simulink library "GRC_Lib"  (R2017b)
settings: Solver=VariableStepAuto  StartTime=0.0  StopTime=10.0  RelTol=1e-3  EnableMultiTasking=on
StartFcn:
  | set_param('AdvancedOperations','ZoomFactor','100');
undefined symbols (not defined in the file): Test
libraries: GRC_Lib x203, simulink x1
(part 1 of 4)
settings Model: Creator=Administrator  LastModifiedBy=WangYunHao
settings DataIOCC: LimitDataPoints=on
settings OptimizationCC: LifeSpan=inf
settings DebuggingCC: AllowSymbolicDim=off  SFUnexpectedBacktrackingDiag=warning  SFNoUnconditionalDefaultTransitionDiag=warning  SFExecutionAtInitializationDiag=none
settings ModelReferenceCC: PropagateSignalLabelsOutOfModel=off
settings CodeAppCC: StateflowObjectComments=on
settings GRTTargetCC: TargetLangStandard=C89/C90 (ANSI)
settings ConfigComp: CovMetricSettings=dw  CovHtmlReporting=on  CovSaveCumulativeToWorkspaceVar=on  CovSaveSingleToWorkspaceVar=on  CovExternalEMLEnable=off

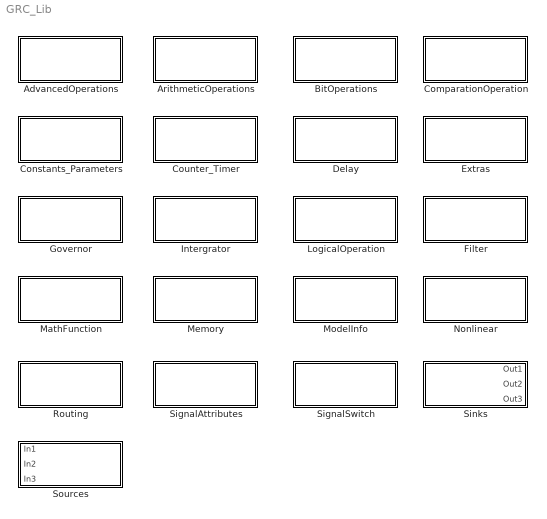
== system GRC_Lib ==
  AdvancedOperations : Subsystem
  ArithmeticOperations : Subsystem
  BitOperations : Subsystem
  ComparationOperation : Subsystem
  Constants_Parameters : Subsystem
  Counter_Timer : Subsystem
  Delay : Subsystem
  Extras : Subsystem
  Filter : Subsystem
  Governor : Subsystem
  Intergrator : Subsystem
  LogicalOperation : Subsystem
  MathFunction : Subsystem
  Memory : Subsystem
  ModelInfo : Subsystem
  Nonlinear : Subsystem
  Routing : Subsystem
  SignalAttributes : Subsystem
  SignalSwitch : Subsystem
  Sinks : Subsystem
  Sources : Subsystem

== system GRC_Lib/AdvancedOperations ==
  note: // What's the 2D length function
      | and lookup methods???
  note: // What's the 1D Length function?
  1D_DynamicLookupTable : Subsystem  TreatAsAtomicUnit=on  mask{method=Use Input Nearest, IpDTx=int8, IpDTy=single, OpDT=single, Length1D=50}
      mask prompts: method "Lookup Method"; IpDTx "xData Datatype"; IpDTy "yData Datatype"; OpDT "Output Data Type"; Length1D "1D Table Length (Min. 2 Max. 200)"
      mask init:
      | %%% Input port number detection 
      | if isequal(str2num(get_param(gcb,'Length1D')),[])
      |     if Length1D<2
      |         error('*** ERROR_11 ***    1D Table Length must belong to [2,200].');
      |     elseif Length1D>200
      |         error('*** ERROR_12 ***    1D Table Length must belong to [2,200].');
      |     else
      |     end
      | else
      |     Lgth = str2num(get_param(gcb,'Length1D'));
      |     if Lgth<2
      |         error('*** ERROR_21 ***    1D Table Length must belong to [2,200].');
      |     elseif Lgth>200
      |         error('*** ERROR_22 ***    1D Table Length must belong to [2,200].');
      |     else
      |     end
      | end
      | 
      | set_param([gcb '/Dynamic1D'],'OutDataTypeStr',OpDT);
      | MethDtr = get_param(gcb,'method');
      | set_param([gcb '/Dynamic1D'], 'LookUpMeth',MethDtr);
      | 
      | DTStry = get_param(gcb,'OpDT');
      | try
      |     if isequal(DTStry,'boolean')
      |         FColor = '[0.901961, 0.313725, 0.078431]'; 
      |     elseif isequal(DTStry,'double')||isequal(DTStry,'single')
      |         FColor = '[0.313725, 0.117647, 0.352941]';  
      |     else
      |         FColor = '[0.196078, 0.549020, 0.549020]';
      |     end        
      | catch
      | end
      | set_param([gcb '/y'],'ForegroundColor',FColor);
      | set_param(gcb,'ForegroundColor',FColor);
      settings: AttributesFormatString=Length = %<Length1D>
      mask TypeOptions method: Interpolation-Use End Values | Use Input Nearest | Use Input Below | Use Input Above
      mask Callback Length1D:
      | % %%% Input port number detection
      | % if isequal(str2num(get_param(gcb,'Length1D')),[])
      | %    error('*** ERROR_1 ***    1D Table Length can not be a %s.',class(get_param(gcb,'Length1D')));
      | % elseif str2num(get_param(gcb,'Length1D'))<2
      | %    error('*** ERROR_2 ***    1D Table Length must belong to [2,200].');
      | % elseif str2num(get_param(gcb,'Length1D'))>200
      | %    error('*** ERROR_2 ***    1D Table Length must belong to [2,200].');
      | % else
      | % end
      mask Display:
      | color('green');
      | disp ('Dynamic\nLookup Table\n(1D)');
  1D_LookupTableContrafunctional : Subsystem
      mask Display:
      | color('green');
      | disp (sprintf('LookupTable\nContrafunctional\n(1D)'));
  2D_DynamicLookupTable : Subsystem  TreatAsAtomicUnit=on  mask{method=Interpolation-Use End Values, Lengthx=10, Lengthy=10, IpDTx=int8, IpDTy=single, IpDTm=int16, MrDT=double, OpDT=double}
      mask prompts: method "Lookup Method"; Lengthx "x Axis Length (Min. 2 Max. 50)"; Lengthy "y Axis Length (Min. 2 Max. 50)"; IpDTx "xData Datatype"; IpDTy "yData Datatype"; IpDTm "mData Datatype"; MrDT "Intermediate Results Data Type"; OpDT "Output Data Type"
      mask init:
      | %%% Input Lentghx number detection
      | if isequal(str2num(get_param(gcb,'Lengthx')),[])
      |     if Lengthx<2
      |         error('*** ERROR_x11 ***    x Axis Length must belong to [2,50].');
      |     elseif Lengthx>50
      |         error('*** ERROR_x12 ***    x Axis Length must belong to [2,50].');
      |     else
      |     end
      | else 
      |     Lgthx = str2num(get_param(gcb,'Lengthx'));
      |     if Lgthx<2
      |         error('*** ERROR_x21 ***    x Axis Length must belong to [2,50].');
      |     elseif Lgthx>50
      |         error('*** ERROR_x22 ***    x Axis Length must belong to [2,50].');
      |     else
      |     end
      | end
      | %%% Input Lentghy number detection
      | if isequal(str2num(get_param(gcb,'Lengthy')),[])
      |     if Lengthy<2
      |         error('*** ERROR_y11 ***    y Axis Length must belong to [2,50].');
      |     elseif Lengthy>50
      |         error('*** ERROR_y12 ***    y Axis Length must belong to [2,50].');
      |     else
      |     end
      | else 
      |     Lgthy = str2num(get_param(gcb,'Lengthy'));
      |     if Lgthy<2
      |         error('*** ERROR_y21 ***    y Axis Length must belong to [2,50].');
      |     elseif Lgthy>50
      |         error('*** ERROR_y22 ***    y Axis Length must belong to [2,50].');
      |     else
      |     end
      | end
      | %%%%%%%%%%%%%%%%%%%%%%%%%%%%%%%%%%%%%%%%%%%%%%%%%%%%%%%%%%%%%%%%%%%%%%%%%%%
      | DTStrM = get_param(gcb,'MrDT');
      | DTStrO = get_param(gcb,'OpDT');
      | set_param([gcb '/Dynamic2D'],'IntermediateResultsDataTypeStr',DTStrM);
      | set_param([gcb '/Dynamic2D'],'OutDataTypeStr',DTStrO);
      | 
      | try
      |     if isequal(DTStrO,'boolean')
      |         FColor = '[0.901961, 0.313725, 0.078431]'; 
      |     elseif isequal(DTStrO,'double')||isequal(DTStrO,'single')
      |         FColor = '[0.313725, 0.117647, 0.352941]';  
      |     else
      |         FColor = '[0.196078, 0.549020, 0.549020]';
      |     end        
      | catch
      | end
      | set_param([gcb '/out'],'ForegroundColor',FColor);
      | set_param(gcb,'ForegroundColor',FColor);
      settings: AttributesFormatString=|
      | xData Length = %<Lengthx>
      | yData Length = %<Lengthy>
      mask TypeOptions method: Interpolation-Use End Values | Use Input Below
      mask Callback Lengthx:
      | % %%% Input port number detection
      | % if isequal(str2num(get_param(gcb,'Lengthx')),[])
      | %    error('*** ERROR_1 ***    x Axis Length can not be a %s.',class(get_param(gcb,'Lengthx')));
      | % elseif str2num(get_param(gcb,'Lengthx'))<2
      | %    error('*** ERROR_2 ***    x Axis Length must belong to [2,50].');
      | % elseif str2num(get_param(gcb,'Lengthx'))>50
      | %    error('*** ERROR_2 ***    x Axis Length must belong to [2,50].');
      | % else
      | % end
      mask Callback Lengthy:
      | % %%% Input port number detection
      | % if isequal(str2num(get_param(gcb,'Lengthy')),[])
      | %    error('*** ERROR_1 ***    y Axis Length can not be a %s.',class(get_param(gcb,'Lengthy')));
      | % elseif str2num(get_param(gcb,'Lengthy'))<2
      | %    error('*** ERROR_2 ***    y Axis Length must belong to [2,50].');
      | % elseif str2num(get_param(gcb,'Lengthy'))>50
      | %    error('*** ERROR_2 ***    y Axis Length must belong to [2,50].');
      | % else
      | % end
      mask Display:
      | color('green');
      | disp (sprintf('Dynamic\nLookup Table\n(2D)'));
  DynAvrgFltr : Subsystem  TreatAsAtomicUnit=on  mask{IpDT=single, RngSizeMsk=5}
      mask prompts: IpDT "Input Data Type"; RngSizeMsk "Dynamic Average Filter Step (Min 1, Max 200)"
      mask init:
      | %%% Input port number detection 
      | if isequal(str2num(get_param(gcb,'RngSizeMsk')),[])
      |     if RngSizeMsk<1
      |         error('*** ERROR_11 ***    Dynamic Average Filter Step must belong to [1,200].');
      |     elseif RngSizeMsk>200
      |         error('*** ERROR_12 ***    Dynamic Average Filter Step must belong to [1,200].');
      |     else
      |     end
      | else
      |     RgSiz = str2num(get_param(gcb,'RngSizeMsk'));
      |     if RgSiz<1
      |         error('*** ERROR_21 ***    Dynamic Average Filter Step must belong to [1,200].');
      |     elseif RgSiz>200
      |         error('*** ERROR_22 ***    Dynamic Average Filter Step must belong to [1,200].');
      |     else
      |     end
      | end
      | 
      | RngSize = RngSizeMsk;
      | DTStr = get_param(gcb,'IpDT');
      | set_param([gcb '/Constant6'],'OutDataTypeStr',DTStr);
      | set_param([gcb '/SUB'],'IpDT',DTStr);
      | set_param([gcb '/DIV'],'IpDT',DTStr);
      | set_param([gcb '/SUM1'],'IpDT',DTStr);
      | 
      | DTStry = get_param([gcb '/SUM1/Sum1'],'OutDataTypeStr');
      | try
      |     if isequal(DTStry,'boolean')
      |         FColor = '[0.901961, 0.313725, 0.078431]'; 
      |     elseif isequal(DTStry,'double')||isequal(DTStry,'single')
      |         FColor = '[0.313725, 0.117647, 0.352941]';  
      |     else
      |         FColor = '[0.196078, 0.549020, 0.549020]';
      |     end        
      | catch
      | end
      | set_param([gcb '/out'],'ForegroundColor',FColor);
      | set_param(gcb,'ForegroundColor',FColor);
      settings: AttributesFormatString=%<RngSizeMsk>
      mask Callback RngSizeMsk:
      | % %%% Input port number detection
      | % if str2num(get_param(gcb,'RngSizeMsk'))<1
      | %    error('*** ERROR ***    Dynamic Average Filter Step must belong to [1,200].');
      | % elseif str2num(get_param(gcb,'RngSizeMsk'))>200
      | %    error('*** ERROR ***    Dynamic Average Filter Step must belong to [1,200].');
      | % else
      | % end
      mask Display:
      | % color('green');
      | % disp ('DynAvrgFltr');
      | image('DynAvrgFltr.jpg');
  VrblTmDelay : Subsystem  TreatAsAtomicUnit=on  mask{IpDTT=double, IpDTu=boolean, MaxBufferMsk=2000, IniVal=0}
      mask prompts: IpDTT "Input T Data Type"; IpDTu "Input u Data Type"; MaxBufferMsk "Maximum Buffer Size (Max 2000)"; IniVal "Initial Value"
      mask init:
      | %%% Input port number detection 
      | if isequal(str2num(get_param(gcb,'MaxBufferMsk')),[])
      |     if MaxBufferMsk<2
      |         error('*** ERROR_11 ***    Maximum Buffer Size must belong to [2,2000].');
      |     elseif MaxBufferMsk>2000
      |         error('*** ERROR_12 ***    Maximum Buffer Size must belong to [2,2000].');
      |     else
      |     end
      | else
      |     MxBf = str2num(get_param(gcb,'MaxBufferMsk'));
      |     if MxBf<2
      |         error('*** ERROR_21 ***    Maximum Buffer Size must belong to [2,2000].');
      |     elseif MxBf>2000
      |         error('*** ERROR_22 ***    Maximum Buffer Size must belong to [2,2000].');
      |     else
      |     end
      | end
      | 
      | MaxBuffer = MaxBufferMsk;
      | initValue = IniVal;
      | DTStrT = get_param(gcb,'IpDTT');
      | set_param([gcb '/Constant'],'OutDataTypeStr',DTStrT);
      | set_param([gcb '/DIV'],'IpDT',DTStrT);
      | 
      | DTStryu = get_param(gcb,'IpDTu');
      | try
      |     if isequal(DTStryu,'boolean')
      |         FColor = '[0.901961, 0.313725, 0.078431]'; 
      |     elseif isequal(DTStryu,'double')||isequal(DTStryu,'single')
      |         FColor = '[0.313725, 0.117647, 0.352941]';  
      |     else
      |         FColor = '[0.196078, 0.549020, 0.549020]';
      |     end        
      | catch
      | end
      | set_param([gcb '/y'],'ForegroundColor',FColor);
      | set_param(gcb,'ForegroundColor',FColor);
      settings: AttributesFormatString=MaxBufferSize = %<MaxBufferMsk>
      mask Callback MaxBufferMsk:
      | % %%% Input port number detection
      | % if str2num(get_param(gcb,'MaxBufferMsk'))<2
      | %    error('*** ERROR ***    Maximum Buffer Size must belong to [2,2000].');
      | % elseif str2num(get_param(gcb,'MaxBufferMsk'))>2000
      | %    error('*** ERROR ***    Maximum Buffer Size must belong to [2,2000].');
      | % else
      | % end
      mask Display:
      | % color('green');
      | % disp ('VrblTmDelay');
      | % image('VrblTmDelay.jpg');
      | image(imread('VrblTmDelay.jpg'),[0.2,0.1,0.7,0.8]);

== system GRC_Lib/ArithmeticOperations ==
  DIV : Subsystem  TreatAsAtomicUnit=on  mask{MinDivVal=1e-15, IpDT=int8}
      mask prompts: MinDivVal "Minimum Allowed Divided Value"; IpDT "Input Data Type"
      mask init:
      | MinVal = MinDivVal;
      | set_param([gcb '/Constant1'],'OutDataTypeStr',IpDT);
      | set_param([gcb '/Divide'],'OutDataTypeStr',IpDT);
      | 
      | DTStry = get_param([gcb '/Divide'],'OutDataTypeStr');
      | try
      |     if isequal(DTStry,'boolean')
      |         FColor = '[0.901961, 0.313725, 0.078431]'; 
      |     elseif isequal(DTStry,'double')||isequal(DTStry,'single')
      |         FColor = '[0.313725, 0.117647, 0.352941]';  
      |     else
      |         FColor = '[0.196078, 0.549020, 0.549020]';
      |     end        
      | catch
      | end
      | set_param([gcb '/Out'],'ForegroundColor',FColor);
      | set_param(gcb,'ForegroundColor',FColor);
      mask Display:
      | color('green');
      | port_label('input',1,'\fontname{Courier New}\fontsize{16}\bf×','texmode','on');
      | port_label('input',2,'\fontname{Courier New}\fontsize{16}\bf÷','texmode','on');
  GAIN : Subsystem  mask(GAIN){K=20, IpDT=double, OFChk=on}
      mask prompts: K "Gain"; IpDT "Input Data Type"; OFChk "Consider Overflow/Underflow (Integers Only)"
      mask help:
      | GRC Library for Function Development
      | (c) GRC, 2016
      |
      | Multiply the input by a gain factor.
      mask init:
      | GAIN=K;
      | 
      | DTStr = get_param(gcb,'IpDT');
      | OFChkStr = get_param(gcb,'OFChk');
      | try
      | if isequal(OFChkStr,'1')
      |     if isequal(DTStr,'int8')||isequal(DTStr,'uint8')
      |         set_param([gcb '/Gain1'],'OutDataTypeStr','uint16'); 
      |     elseif isequal(DTStr,'int16')||isequal(DTStr,'uint16')
      |         set_param([gcb '/Gain1'],'OutDataTypeStr','uint32'); 
      |     elseif isequal(DTStr,'int32')||isequal(DTStr,'uint32')
      |         set_param([gcb '/Gain1'],'OutDataTypeStr','uint32'); 
      |     elseif isequal(DTStr,'double')
      |         set_param([gcb '/Gain1'],'OutDataTypeStr','double'); 
      |     elseif isequal(DTStr,'single')
      |         set_param([gcb '/Gain1'],'OutDataTypeStr','single');
      |     end
      | else
      |     set_param([gcb '/Gain1'],'OutDataTypeStr',DTStr);
      | end
      | catch
      | end
      | 
      | DTStry = get_param([gcb '/Gain1'],'OutDataTypeStr');
      | try
      |     if isequal(DTStry,'boolean')
      |         FColor = '[0.901961, 0.313725, 0.078431]'; 
      |     elseif isequal(DTStry,'double')||isequal(DTStry,'single')
      |         FColor = '[0.313725, 0.117647, 0.352941]';  
      |     else
      |         FColor = '[0.196078, 0.549020, 0.549020]';
      |     end        
      | catch
      | end
      | set_param([gcb '/Out1'],'ForegroundColor',FColor);
      | set_param(gcb,'ForegroundColor',FColor);
      settings: AttributesFormatString=K=%<K>
      mask Display:
      | color('green');
      | disp('\fontsize{10}\bfK','texmode','on');
  MUL : Subsystem  mask(MUL){IpDT=double, OFChk=on}
      mask prompts: IpDT "Input Data Type"; OFChk "Consider Overflow/Underflow (Integers Only)"
      mask help:
      | GRC Library for Function Development
      | (c) GRC, 2016
      |
      | Multiplies two inputs.
      mask init:
      | DTStr = get_param(gcb,'IpDT');
      | OFChkStr = get_param(gcb,'OFChk');
      | try
      | if isequal(OFChkStr,'1')
      |     if isequal(DTStr,'int8')||isequal(DTStr,'uint8')
      |         set_param([gcb '/Mul1'],'OutDataTypeStr','uint16'); 
      |     elseif isequal(DTStr,'int16')||isequal(DTStr,'uint16')
      |         set_param([gcb '/Mul1'],'OutDataTypeStr','uint32'); 
      |     elseif isequal(DTStr,'int32')||isequal(DTStr,'uint32')
      |         set_param([gcb '/Mul1'],'OutDataTypeStr','uint32'); 
      |     elseif isequal(DTStr,'double')
      |         set_param([gcb '/Mul1'],'OutDataTypeStr','double'); 
      |     elseif isequal(DTStr,'single')
      |         set_param([gcb '/Mul1'],'OutDataTypeStr','single');
      |     end
      | else
      |     set_param([gcb '/Mul1'],'OutDataTypeStr',DTStr);
      | end
      | catch
      | end
      | 
      | DTStry = get_param([gcb '/Mul1'],'OutDataTypeStr');
      | try
      |     if isequal(DTStry,'boolean')
      |         FColor = '[0.901961, 0.313725, 0.078431]'; 
      |     elseif isequal(DTStry,'double')||isequal(DTStry,'single')
      |         FColor = '[0.313725, 0.117647, 0.352941]';  
      |     else
      |         FColor = '[0.196078, 0.549020, 0.549020]';
      |     end        
      | catch
      | end
      | set_param([gcb '/Out1'],'ForegroundColor',FColor);
      | set_param(gcb,'ForegroundColor',FColor);
      mask Display:
      | color('green');
      | disp('\fontsize{14}\bf×','texmode','on');
  NEG : Subsystem  mask(NEG){DTNEG=double}
      mask prompts: DTNEG "Output Data Type"
      mask help:
      | GRC Library for Function Development
      | (c) GRC, 2016
      |
      | Negates the input signal.
      mask init:
      | dtneg=get_param(gcb,'DTNEG');
      | set_param([gcb '/Neg1'],'OutDataTypeStr',dtneg);
      | 
      | DTStry = get_param([gcb '/Neg1'],'OutDataTypeStr');
      | try
      |     if isequal(DTStry,'boolean')
      |         FColor = '[0.901961, 0.313725, 0.078431]'; 
      |     elseif isequal(DTStry,'double')||isequal(DTStry,'single')
      |         FColor = '[0.313725, 0.117647, 0.352941]';  
      |     else
      |         FColor = '[0.196078, 0.549020, 0.549020]';
      |     end        
      | catch
      | end
      | set_param([gcb '/Out1'],'ForegroundColor',FColor);
      | set_param(gcb,'ForegroundColor',FColor);
      mask Display:
      | color('green')
      | disp('\fontsize{10}\bf-1','texmode','on')
  SUB : Subsystem  mask(SUB){IpDT=double, OFChk=on}
      mask prompts: IpDT "Input Data Type"; OFChk "Consider Overflow/Underflow (Integers Only)"
      mask help:
      | GRC Library for Function Development
      | (c) GRC, 2016
      |
      | Subtract input 2 from input 1.
      |
      | Input must have the same data type.
      mask init:
      | DTStr = get_param(gcb,'IpDT');
      | OFChkStr = get_param(gcb,'OFChk');
      | try
      | if isequal(OFChkStr,'1')
      |     if isequal(DTStr,'int8')||isequal(DTStr,'uint8')
      |         set_param([gcb '/Sub1'],'OutDataTypeStr','uint16'); 
      |     elseif isequal(DTStr,'int16')||isequal(DTStr,'uint16')
      |         set_param([gcb '/Sub1'],'OutDataTypeStr','uint32'); 
      |     elseif isequal(DTStr,'int32')||isequal(DTStr,'uint32')
      |         set_param([gcb '/Sub1'],'OutDataTypeStr','uint32'); 
      |     elseif isequal(DTStr,'double')
      |         set_param([gcb '/Sub1'],'OutDataTypeStr','double'); 
      |     elseif isequal(DTStr,'single')
      |         set_param([gcb '/Sub1'],'OutDataTypeStr','single');
      |     end
      | else
      |     set_param([gcb '/Sub1'],'OutDataTypeStr',DTStr);
      | end
      | catch
      | end
      | 
      | DTStry = get_param([gcb '/Sub1'],'OutDataTypeStr');
      | try
      |     if isequal(DTStry,'boolean')
      |         FColor = '[0.901961, 0.313725, 0.078431]'; 
      |     elseif isequal(DTStry,'double')||isequal(DTStry,'single')
      |         FColor = '[0.313725, 0.117647, 0.352941]';  
      |     else
      |         FColor = '[0.196078, 0.549020, 0.549020]';
      |     end        
      | catch
      | end
      | set_param([gcb '/Out1'],'ForegroundColor',FColor);
      | set_param(gcb,'ForegroundColor',FColor);
      mask Display:
      | color('green');
      | port_label('input',1,'\fontname{Courier New}\fontsize{16}\bf+','texmode','on');
      | port_label('input',2,'\fontname{Courier New}\fontsize{16}\bf-','texmode','on');
  SUB_Uint : Subsystem  TreatAsAtomicUnit=on  mask{IpDT=uint8}
      mask prompts: IpDT "Input Data Type"
      mask init:
      | DTStr = get_param(gcb,'IpDT');
      | set_param([gcb '/Constant'],'OutDataTypeStr',DTStr);
      | 
      | DTStry = get_param([gcb '/Constant'],'OutDataTypeStr');
      | try
      |     if isequal(DTStry,'boolean')
      |         FColor = '[0.901961, 0.313725, 0.078431]'; 
      |     elseif isequal(DTStry,'double')||isequal(DTStry,'single')
      |         FColor = '[0.313725, 0.117647, 0.352941]';  
      |     else
      |         FColor = '[0.196078, 0.549020, 0.549020]';
      |     end        
      | catch
      | end
      | set_param([gcb '/Out'],'ForegroundColor',FColor);
      | set_param(gcb,'ForegroundColor',FColor);
      settings: AttributesFormatString=SUB_Uint
      mask Display:
      | color('blue');
      | port_label('input',1,'\fontname{Courier New}\fontsize{16}\bf+','texmode','on');
      | port_label('input',2,'\fontname{Courier New}\fontsize{16}\bf-','texmode','on');
  SUM : Subsystem  mask(SUM){IpDT=single, OFChk=on}
      mask prompts: IpDT "Input Data Type"; OFChk "Consider Overflow/Underflow (Integers Only)"
      mask help:
      | GRC Library for Function Development
      | (c) GRC, 2016
      |
      | Caculates the sum of two input values.
      |
      | Input must have the same data type.
      mask init:
      | DTStr = get_param(gcb,'IpDT');
      | OFChkStr = get_param(gcb,'OFChk');
      | try
      | if isequal(OFChkStr,'1')
      |     if isequal(DTStr,'int8')||isequal(DTStr,'uint8')
      |         set_param([gcb '/Sum1'],'OutDataTypeStr','uint16');
      |     elseif isequal(DTStr,'int16')||isequal(DTStr,'uint16')
      |         set_param([gcb '/Sum1'],'OutDataTypeStr','uint32');
      |     elseif isequal(DTStr,'int32')||isequal(DTStr,'uint32')
      |         set_param([gcb '/Sum1'],'OutDataTypeStr','uint32'); 
      |     elseif isequal(DTStr,'double')
      |         set_param([gcb '/Sum1'],'OutDataTypeStr','double'); 
      |     elseif isequal(DTStr,'single')
      |         set_param([gcb '/Sum1'],'OutDataTypeStr','single');
      |     end
      | else
      |     set_param([gcb '/Sum1'],'OutDataTypeStr',DTStr);
      | end
      | catch
      | end
      | 
      | DTStry = get_param([gcb '/Sum1'],'OutDataTypeStr');
      | try
      |     if isequal(DTStry,'boolean')
      |         FColor = '[0.901961, 0.313725, 0.078431]'; 
      |     elseif isequal(DTStry,'double')||isequal(DTStry,'single')
      |         FColor = '[0.313725, 0.117647, 0.352941]';  
      |     else
      |         FColor = '[0.196078, 0.549020, 0.549020]';
      |     end        
      | catch
      | end
      | set_param([gcb '/Out1'],'ForegroundColor',FColor);
      | set_param(gcb,'ForegroundColor',FColor);
      mask Display:
      | color('green')
      | port_label('input',1,'\fontname{Courier New}\fontsize{16}\bf+','texmode','on')
      | port_label('input',2,'\fontname{Courier New}\fontsize{16}\bf+','texmode','on')

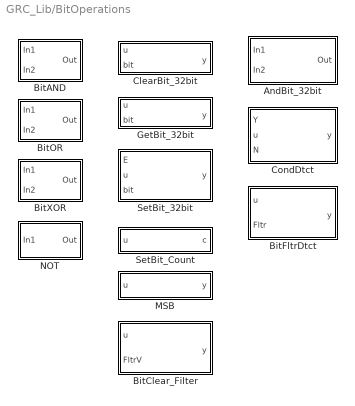
== system GRC_Lib/BitOperations ==
  AndBit_32bit : Subsystem  TreatAsAtomicUnit=on
      mask help:
      | This block judge whether at least one bit is set or not. If any bits are set, output is boolean 1, otherwise output is boolean 0.
      |
      | input 1 and input 2 should have same data type, and output is boolean.
      mask init:
      | FColor = '[0.901961, 0.313725, 0.078431]'; 
      | try
      |     set_param([gcb '/Out'],'ForegroundColor',FColor);
      |     set_param(gcb,'ForegroundColor',FColor);
      | catch
      | end
      mask Display:
      | % color('red');
      | % disp ('AndBit\n(8|16|32bit)');
      | image(imread('AndBit_32bit.jpg'),[0.03,0.1,0.95,0.8]);
  BitAND : Subsystem  TreatAsAtomicUnit=on  mask{IpDT=uint8}
      mask prompts: IpDT "Input Data Type"
      mask init:
      | % set_param([gcb '/Chart/Out'],'OutDataTypeStr',IpDT);
      | % set_param([gcb '/Out'],'OutDataTypeStr',IpDT);
      | % set_param([gcb '/In1'],'OutDataTypeStr',IpDT);
      | % set_param([gcb '/In2'],'OutDataTypeStr',IpDT);
      mask Callback IpDT:
      | try
      | set_param([gcb '/Out'],'OutDataTypeStr',IpDT);
      | catch
      | end
      mask Display:
      | color('green');
      | disp ('Bitwise\n(AND)');
  BitClear_Filter : Subsystem  TreatAsAtomicUnit=on  mask{IpDT=uint32}
      mask prompts: IpDT "Input Data Type"
      mask init:
      | % DTStr = get_param(gcb,'IpDT');
      | % set_param([gcb '/y'],'OutDataTypeStr',DTStr); 
      | 
      | FColor = '[0.196078, 0.549020, 0.549020]'; 
      | try
      |     set_param([gcb '/y'],'ForegroundColor',FColor);
      |     set_param(gcb,'ForegroundColor',FColor);
      | catch
      | end
      mask Display:
      | % color('blue');
      | % disp ('BitClear_Fltr\n(8|16|32bit)');
      | image(imread('BitClear_Filter.jpg'),[0.1,0.1,0.8,0.9]);
  BitFltrDtct : Subsystem  TreatAsAtomicUnit=on  mask{IpDT=uint32}
      mask prompts: IpDT "Input Data Type"
      mask init:
      | DTStr = get_param(gcb,'IpDT');
      | set_param([gcb '/BitAND'],'IpDT',DTStr);
      | 
      | FColor = '[0.901961, 0.313725, 0.078431]'; 
      | try
      |     set_param([gcb '/y'],'ForegroundColor',FColor);
      |     set_param(gcb,'ForegroundColor',FColor);
      | catch
      | end
      mask Display:
      | % color('red');
      | % disp ('BitFltrDtct\n(8|16|32bit)');
      | image(imread('BitFltrDtct.jpg'),[0.1,0.1,0.8,0.9]);
  BitOR : Subsystem  TreatAsAtomicUnit=on  mask{IpDT=uint8}
      mask prompts: IpDT "Input Data Type"
      mask init:
      | % set_param([gcb '/Chart/Out'],'OutDataTypeStr',IpDT);
      | % set_param([gcb '/Out'],'OutDataTypeStr',IpDT);
      | % set_param([gcb '/In1'],'OutDataTypeStr',IpDT);
      | % set_param([gcb '/In2'],'OutDataTypeStr',IpDT);
      mask Display:
      | color('green');
      | disp ('Bitwise\n(OR)');
  BitXOR : Subsystem  TreatAsAtomicUnit=on  mask{IpDT=uint8}
      mask prompts: IpDT "Input Data Type"
      mask init: same as GRC_Lib/BitOperations/BitOR
      mask Display:
      | color('green');
      | disp ('Bitwise\n(XOR)');
  ClearBit_32bit : Subsystem  TreatAsAtomicUnit=on  mask{OpDT=uint32, dataLength=32, msbClearFlag=2147483647}
      mask prompts: OpDT "Output Data Type"; dataLength "Data Type Length"; msbClearFlag "MSB Clear Flag Value"
      mask help:
      | Sets the bit at position "bit" of input value "u" to zero.
      |
      | Position value(bit) data type mast be uint8, and input u supports 8-bit, 16-bit and 32-bit unsigned integer values.
      mask init:
      | DTStr = get_param(gcb,'OpDT');
      | set_param([gcb '/One'],'OutDataTypeStr',DTStr); 
      | set_param([gcb '/msb_clear_flag'],'OutDataTypeStr',DTStr); 
      | 
      | try
      |     if isequal(DTStr,'uint32')
      |         dataLength = 32; 
      |         msbClearFlag = 2147483647;
      |     elseif isequal(DTStr,'uint16')
      |         dataLength = 16; 
      |         msbClearFlag = 32767;
      |     elseif isequal(DTStr,'uint8')
      |         dataLength = 8; 
      |         msbClearFlag = 127;
      |     else
      | end
      | catch
      | end
      | 
      | DTStry = get_param([gcb '/msb_clear_flag'],'OutDataTypeStr');
      | try
      |     if isequal(DTStry,'boolean')
      |         FColor = '[0.901961, 0.313725, 0.078431]'; 
      |     elseif isequal(DTStry,'double')||isequal(DTStry,'single')
      |         FColor = '[0.313725, 0.117647, 0.352941]';  
      |     else
      |         FColor = '[0.196078, 0.549020, 0.549020]';
      |     end        
      | catch
      | end
      | set_param([gcb '/y'],'ForegroundColor',FColor);
      | set_param(gcb,'ForegroundColor',FColor);
      mask Display:
      | % color('blue');
      | % disp ('ClearBit\n(8|16|32bit)');
      | image(imread('ClearBit_32bit.jpg'),[0.1,0.1,0.8,0.7]);
  CondDtct : Subsystem  TreatAsAtomicUnit=on  mask{IpDT=uint8}
      mask prompts: IpDT "Input Data Type"
      mask init:
      | DTStr = get_param(gcb,'IpDT');
      | set_param([gcb '/BitAND'],'IpDT',DTStr); 
      | set_param([gcb '/BitAND1'],'IpDT',DTStr); 
      | set_param([gcb '/BitXOR'],'IpDT',DTStr);
      | 
      | FColor = '[0.901961, 0.313725, 0.078431]'; 
      | try
      |     set_param([gcb '/y'],'ForegroundColor',FColor);
      |     set_param(gcb,'ForegroundColor',FColor);
      | catch
      | end
      mask Display:
      | % color('red');
      | % disp ('CondDtct\n(8|16|32bit)');
      | image(imread('CondDtct.jpg'),[0.1,0.1,0.82,0.83]);
  GetBit_32bit : Subsystem  TreatAsAtomicUnit=on  mask{IpDT=uint16, datalength=32}
      mask prompts: IpDT "Input Data Type"; datalength "Data Type Length"
      mask init:
      | DTStr = get_param(gcb,'IpDT');
      | try
      |     if isequal(DTStr,'uint32')
      |         datalength = 32; 
      |     elseif isequal(DTStr,'uint16')
      |         datalength = 16; 
      |     elseif isequal(DTStr,'uint8')
      |         datalength = 8; 
      |     else
      | end
      | catch
      | end
      mask Display:
      | % color('blue');
      | % disp ('GetBit\n(8|16|32bit)');
      | image(imread('GetBit_32bit.jpg'),[0.1,0.1,0.8,0.7]);
  MSB : Subsystem  TreatAsAtomicUnit=on  mask{IpDT=uint32, IniIdx=4}
      mask prompts: IpDT "Input Data Type"; IniIdx "Initial Index"
      mask init:
      | DTStr = get_param(gcb,'IpDT');
      | 
      | try
      |     if isequal(DTStr,'uint32')
      |         IniIdx = 4;
      |     elseif isequal(DTStr,'uint16')
      |         IniIdx = 3;
      |     elseif isequal(DTStr,'uint8')
      |         IniIdx = 2;
      |     else
      | end
      | catch
      | end
      | 
      | FColor = '[0.196078, 0.549020, 0.549020]'; 
      | try
      |     set_param([gcb '/y'],'ForegroundColor',FColor);
      |     set_param(gcb,'ForegroundColor',FColor);
      | catch
      | end
      mask Display:
      | % color('blue');
      | % disp ('MSB\n(8|16|32bit)');
      | image(imread('MSB.jpg'),[0.05,0.2,0.95,0.6]);
  NOT : Subsystem  TreatAsAtomicUnit=on  mask{IpDT=uint8}
      mask prompts: IpDT "Input Data Type"
      mask init:
      | % set_param([gcb '/Out'],'OutDataTypeStr',IpDT);
      | % set_param([gcb '/In1'],'OutDataTypeStr',IpDT);
      | % set_param([gcb '/Chart/Out'],'OutDataTypeStr',IpDT);
      mask Display:
      | color('green');
      | disp ('Bitwise\n(NOT)');
  SetBit_32bit : Subsystem  TreatAsAtomicUnit=on  mask{IpDT=uint32, datalength=32, msbSetFlag=2147483648}
      mask prompts: IpDT "Input Data Type"; datalength "Data Type Length"; msbSetFlag "MSB Clear Flag Value"
      mask help:
      | Sets the bit at position "bit" of input value "u" to one if enable E is true, and keep others bits, then output to y. If E is false, output u to y directly.
      |
      | Position value(bit) data type mast be uint8, and input u supports 8-bit, 16-bit and 32-bit unsigned integer values.
      mask init:
      | DTStr = get_param(gcb,'IpDT');
      | set_param([gcb '/msb_set_flag'],'OutDataTypeStr',DTStr); 
      | 
      | try
      |     if isequal(DTStr,'uint32')
      |         datalength = 32; 
      |         msbSetFlag = 2147483648;
      |     elseif isequal(DTStr,'uint16')
      |         datalength = 16; 
      |         msbSetFlag = 32767;
      |     elseif isequal(DTStr,'uint8')
      |         datalength = 8; 
      |         msbSetFlag = 127;
      |     else
      | end
      | catch
      | end
      | 
      | DTStry = get_param(gcb,'IpDT');
      | try
      |     if isequal(DTStry,'boolean')
      |         FColor = '[0.901961, 0.313725, 0.078431]'; 
      |     elseif isequal(DTStry,'double')||isequal(DTStry,'single')
      |         FColor = '[0.313725, 0.117647, 0.352941]';  
      |     else
      |         FColor = '[0.196078, 0.549020, 0.549020]';
      |     end        
      | catch
      | end
      | set_param([gcb '/y'],'ForegroundColor',FColor);
      | set_param(gcb,'ForegroundColor',FColor);
      mask Display:
      | % color('blue');
      | % disp ('SetBit\n(8|16|32bit)');
      | image(imread('SetBit_32bit.jpg'),[0.1,0.05,0.8,0.88]);
  SetBit_Count : Subsystem  TreatAsAtomicUnit=on  mask{IpDT=uint32}
      mask prompts: IpDT "Input Data Type"
      mask init:
      | FColor = '[0.196078, 0.549020, 0.549020]';
      | try
      |     set_param([gcb '/c'],'ForegroundColor',FColor);
      |     set_param(gcb,'ForegroundColor',FColor);
      | catch
      | end
      mask Display:
      | % color('green');
      | % disp ('SetBitCount\n(8|16|32bit)');
      | image(imread('SetBit_Count.jpg'),[0.05,0.2,0.95,0.6]);

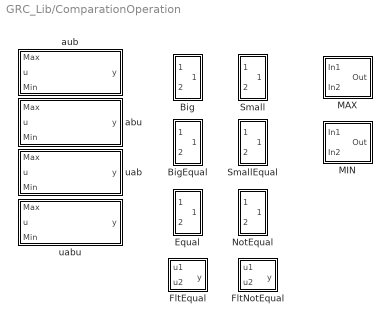
== system GRC_Lib/ComparationOperation ==
  Big : Subsystem  mask{IpDT=double}
      mask prompts: IpDT "Input Data Type"
      mask init:
      | FColor = '[0.901961, 0.313725, 0.078431]'; 
      | try
      |     set_param([gcb '/y'],'ForegroundColor',FColor);
      |     set_param(gcb,'ForegroundColor',FColor);
      | catch
      | end
      mask Display:
      | color('green');
      | disp('\bf>','texmode','on');
  BigEqual : Subsystem  mask{IpDT=double}
      mask prompts: IpDT "Input Data Type"
      mask init:
      | % set_param([gcb '/u1'],'OutDataTypeStr',IpDT);
      | % set_param([gcb '/u2'],'OutDataTypeStr',IpDT);
      | 
      | FColor = '[0.901961, 0.313725, 0.078431]'; 
      | try
      |     set_param([gcb '/y'],'ForegroundColor',FColor);
      |     set_param(gcb,'ForegroundColor',FColor);
      | catch
      | end
      mask Display:
      | color('green');
      | disp('\bf>=','texmode','on');
  Equal : Subsystem  mask{IpDT=double}
      mask prompts: IpDT "Input Data Type"
      mask init: same as GRC_Lib/ComparationOperation/BigEqual
      mask Display:
      | color('green');
      | disp('\bf==','texmode','on');
  FltEqual : Subsystem  TreatAsAtomicUnit=on  mask{OpDT=single, Eplison=1e-15}
      mask prompts: OpDT "Output Data Type"; Eplison "Error Range"
      mask init:
      | err = Eplison;
      | % set_param([gcb '/MIN'],'OpDT',OpDT);
      | set_param([gcb '/Epslion'],'OutDataTypeStr',OpDT);
      | 
      | 
      | FColor = '[0.901961, 0.313725, 0.078431]'; 
      | try
      |     set_param([gcb '/y'],'ForegroundColor',FColor);
      |     set_param(gcb,'ForegroundColor',FColor);
      | catch
      | end
      mask Display:
      | color('green');
      | disp (sprintf('Float\n=='));
  FltNotEqual : Subsystem  TreatAsAtomicUnit=on  mask{OpDT=double, Eplison=1e-15}
      mask prompts: OpDT "Output Data Type"; Eplison "Error Range"
      mask init:
      | err = Eplison;
      | % set_param([gcb '/MIN'],'OpDT',OpDT);
      | set_param([gcb '/Epslion'],'OutDataTypeStr',OpDT);
      | 
      | FColor = '[0.901961, 0.313725, 0.078431]'; 
      | try
      |     set_param([gcb '/y'],'ForegroundColor',FColor);
      |     set_param(gcb,'ForegroundColor',FColor);
      | catch
      | end
      mask Display:
      | color('green');
      | disp (sprintf('Float\n~='));
  MAX : Subsystem  TreatAsAtomicUnit=on  mask{OpDT=int32}
      mask prompts: OpDT "Output Data Type"
      mask init:
      | % set_param([gcb '/SWT2'],'OpDT',OpDT);
      | % set_param([gcb '/Out'],'OutDataTypeStr',OpDT);
      mask Display:
      | color('green');
      | disp('MAX','texmode','on');
  MIN : Subsystem  TreatAsAtomicUnit=on  mask{OpDT=double}
      mask prompts: OpDT "Output Data Type"
      mask init:
      | % set_param([gcb '/SWT2'],'OpDT',OpDT);
      | % set_param([gcb '/Out'],'OutDataTypeStr',OpDT);
      mask Display:
      | color('green');
      | disp('MIN','texmode','on');
  NotEqual : Subsystem  mask{IpDT=double}
      mask prompts: IpDT "Input Data Type"
      mask init: same as GRC_Lib/ComparationOperation/BigEqual
      mask Display:
      | color('green');
      | disp('\bf~=','texmode','on');
  Small : Subsystem  mask{IpDT=double}
      mask prompts: IpDT "Input Data Type"
      mask init:
      | FColor = '[0.901961, 0.313725, 0.078431]'; 
      | try
      |     set_param([gcb '/y'],'ForegroundColor',FColor);
      |     set_param(gcb,'ForegroundColor',FColor);
      | catch
      | end
      mask Display:
      | color('green');
      | disp('\bf<','texmode','on');
  SmallEqual : Subsystem  mask{IpDT=double}
      mask prompts: IpDT "Input Data Type"
      mask init: same as GRC_Lib/ComparationOperation/BigEqual
      mask Display:
      | color('green');
      | disp('\bf<=','texmode','on');
  abu : Subsystem  mask{IpDT=double}
      mask prompts: IpDT "Input Data Type"
      mask init:
      | % set_param([gcb '/Max'],'OutDataTypeStr',IpDT);
      | % set_param([gcb '/Min'],'OutDataTypeStr',IpDT);
      | % set_param([gcb '/u'],'OutDataTypeStr',IpDT);
      | 
      | FColor = '[0.901961, 0.313725, 0.078431]'; 
      | try
      |     set_param([gcb '/y'],'ForegroundColor',FColor);
      |     set_param(gcb,'ForegroundColor',FColor);
      | catch
      | end
      mask Display:
      | color('green');
      | disp('\bfu ∈ [a,b)','texmode','on');
  aub : Subsystem  mask{IpDT=uint8}
      mask prompts: IpDT "Input Data Type"
      mask init: same as GRC_Lib/ComparationOperation/abu
      mask Display:
      | color('green');
      | disp('\bfu ∈ [a,b]','texmode','on');
  uab : Subsystem  mask{IpDT=double}
      mask prompts: IpDT "Input Data Type"
      mask init: same as GRC_Lib/ComparationOperation/abu
      mask Display:
      | color('green');
      | disp('\bfu ∈ (a,b]','texmode','on');
  uabu : Subsystem  mask{IpDT=double}
      mask prompts: IpDT "Input Data Type"
      mask init: same as GRC_Lib/ComparationOperation/abu
      mask Display:
      | color('green');
      | disp('\bfu ∈ (a,b)','texmode','on');
